simulink model "polyval_test_tmp"  (Simulink 8.3)
settings: Solver=ode45  StartTime=0.0  StopTime=10.0  RelTol=1e-3
settings Model: Creator=arnaud  LastModifiedBy=hbourbou
settings DataIOCC: SaveFormat=StructureWithTime
settings OptimizationCC: ExpressionDepthLimit=2147483647
settings DebuggingCC: FcnCallInpInsideContextMsg=EnableAllAsWarning  FrameProcessingCompatibilityMsg=error

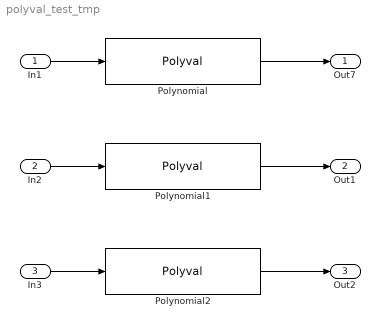
== system polyval_test_tmp ==
  In1 : Inport  PortDimensions=1
  In2 : Inport  Port=2  PortDimensions=3
  In3 : Inport  Port=3  PortDimensions=[2 3]
  Polynomial : Polyval  Coefs=[ 3, 2, -10 ]
  Polynomial1 : Polyval  Coefs=[ 3, 2.5e-006, -10 ]
  Polynomial2 : Polyval  Coefs=[ -15.8, .5e-15, -10 ]
  Out7 : Outport
  Out1 : Outport  Port=2
  Out2 : Outport  Port=3
  wires:
  In1/1 -> Polynomial/1
  Polynomial/1 -> Out7/1
  In2/1 -> Polynomial1/1
  Polynomial1/1 -> Out1/1
  In3/1 -> Polynomial2/1
  Polynomial2/1 -> Out2/1
